simulink model "MINI_upgrade"  (R2021a)
settings: Solver=FixedStepAuto  StartTime=0.0  StopTime=10.0  FixedStep=0.001  RelTol=1e-3
InitFcn:
  | parameters;
model workspace: external: MATLAB File .\MINI_upgrade_DataFile.m (data not in the file)
values from neighbouring files (symbols this model uses):
  th10_ofst = -pi    (= -3.14159265359)    [parameters.m]
  th11_ofst = 0    [parameters.m]
  th12_ofst = pi    (= 3.14159265359)    [parameters.m]
  th13_ofst = 0    [parameters.m]
  th14_ofst = 0    [parameters.m]
  th15_ofst = 0    [parameters.m]
  th16_ofst = 0    [parameters.m]
  th1_ofst = pi/2    (= 1.57079632679)    [parameters.m]
  th2_ofst = -pi/2    (= -1.57079632679)    [parameters.m]
  th3_ofst = pi/2    (= 1.57079632679)    [parameters.m]
  th4_ofst = pi/2    (= 1.57079632679)    [parameters.m]
  th5_ofst = 0    [parameters.m]
  th6_ofst = 0    [parameters.m]
  th7_ofst = pi/2    (= 1.57079632679)    [parameters.m]
  th8_ofst = pi/2    (= 1.57079632679)    [parameters.m]
  th9_ofst = 0    [parameters.m]
undefined symbols (not defined in the file or in its folder): smiData, X, Y, Z
libraries: sm_lib x484, nesl_utility x17
(part 9 of 9)

== system MINI_upgrade/Upgraded_Body_1_RIGID/Copy_of_Upgraded_BodyUpgraded_Body_1_RIGID/Rivet_2_RIGID/River_01_1_RIGID ==
  ReferenceFrame : sm_lib/Frames and Transforms/Reference Frame
  Solid : sm_lib/Body Elements/File Solid  ExtGeomFileName=River_01_Default_sldprt.STEP  UnitType=FromFile  ExtGeomFileUnits=m  StepReaderType=HEX  ExportConvexHullGeometry=off  InertiaType=Custom  Mass=smiData.Solid(11).mass  MassUnits=kg  CenterOfMass=smiData.Solid(11).CoM  CenterOfMassUnits=mm  MomentsOfInertia=smiData.Solid(11).MoI  MomentsOfInertiaUnits=kg*mm^2  ProductsOfInertia=smiData.Solid(11).PoI  ProductsOfInertiaUnits=kg*mm^2  BasedOnType=DensityFromFile  Density=1000  DensityUnits=kg/m^3  DoExposeReferenceFrame=on  SerializedFrames=<Frames/>  GraphicType=FromGeometry  MarkerShape=Sphere  MarkerSize=10  GraphicVisPropType=SimpleVisualProperties  GraphicDiffuseColor=smiData.Solid(11).color  GraphicSpecularColor=[0.5 0.5 0.5 1.0]  GraphicAmbientColor=[0.15 0.15 0.15 1.0]  GraphicEmissiveColor=[0.0 0.0 0.0 1.0]  GraphicShininess=75  GraphicOpacity=smiData.Solid(11).opacity
  F : PMIOPort  Side=Left
  connections:
  Solid/RConn1 -- ReferenceFrame/RConn1 -- F/RConn1

== system MINI_upgrade/Upgraded_Body_1_RIGID/Copy_of_Upgraded_BodyUpgraded_Body_1_RIGID/Rivet_2_RIGID/River_02_1_RIGID ==
  ReferenceFrame : sm_lib/Frames and Transforms/Reference Frame
  Solid : sm_lib/Body Elements/File Solid  ExtGeomFileName=River_02_Default_sldprt.STEP  UnitType=FromFile  ExtGeomFileUnits=m  StepReaderType=HEX  ExportConvexHullGeometry=off  InertiaType=Custom  Mass=smiData.Solid(12).mass  MassUnits=kg  CenterOfMass=smiData.Solid(12).CoM  CenterOfMassUnits=mm  MomentsOfInertia=smiData.Solid(12).MoI  MomentsOfInertiaUnits=kg*mm^2  ProductsOfInertia=smiData.Solid(12).PoI  ProductsOfInertiaUnits=kg*mm^2  BasedOnType=DensityFromFile  Density=1000  DensityUnits=kg/m^3  DoExposeReferenceFrame=on  SerializedFrames=<Frames/>  GraphicType=FromGeometry  MarkerShape=Sphere  MarkerSize=10  GraphicVisPropType=SimpleVisualProperties  GraphicDiffuseColor=smiData.Solid(12).color  GraphicSpecularColor=[0.5 0.5 0.5 1.0]  GraphicAmbientColor=[0.15 0.15 0.15 1.0]  GraphicEmissiveColor=[0.0 0.0 0.0 1.0]  GraphicShininess=75  GraphicOpacity=smiData.Solid(12).opacity
  F : PMIOPort  Side=Left
  connections:
  Solid/RConn1 -- ReferenceFrame/RConn1 -- F/RConn1

== system MINI_upgrade/Upgraded_Body_1_RIGID/Copy_of_Upgraded_BodyUpgraded_Body_1_RIGID/Rivet_3_RIGID/River_01_1_RIGID ==
  ReferenceFrame : sm_lib/Frames and Transforms/Reference Frame
  Solid : sm_lib/Body Elements/File Solid  ExtGeomFileName=River_01_Default_sldprt.STEP  UnitType=FromFile  ExtGeomFileUnits=m  StepReaderType=HEX  ExportConvexHullGeometry=off  InertiaType=Custom  Mass=smiData.Solid(11).mass  MassUnits=kg  CenterOfMass=smiData.Solid(11).CoM  CenterOfMassUnits=mm  MomentsOfInertia=smiData.Solid(11).MoI  MomentsOfInertiaUnits=kg*mm^2  ProductsOfInertia=smiData.Solid(11).PoI  ProductsOfInertiaUnits=kg*mm^2  BasedOnType=DensityFromFile  Density=1000  DensityUnits=kg/m^3  DoExposeReferenceFrame=on  SerializedFrames=<Frames/>  GraphicType=FromGeometry  MarkerShape=Sphere  MarkerSize=10  GraphicVisPropType=SimpleVisualProperties  GraphicDiffuseColor=smiData.Solid(11).color  GraphicSpecularColor=[0.5 0.5 0.5 1.0]  GraphicAmbientColor=[0.15 0.15 0.15 1.0]  GraphicEmissiveColor=[0.0 0.0 0.0 1.0]  GraphicShininess=75  GraphicOpacity=smiData.Solid(11).opacity
  F : PMIOPort  Side=Left
  connections:
  Solid/RConn1 -- ReferenceFrame/RConn1 -- F/RConn1

== system MINI_upgrade/Upgraded_Body_1_RIGID/Copy_of_Upgraded_BodyUpgraded_Body_1_RIGID/Rivet_3_RIGID/River_02_1_RIGID ==
  ReferenceFrame : sm_lib/Frames and Transforms/Reference Frame
  Solid : sm_lib/Body Elements/File Solid  ExtGeomFileName=River_02_Default_sldprt.STEP  UnitType=FromFile  ExtGeomFileUnits=m  StepReaderType=HEX  ExportConvexHullGeometry=off  InertiaType=Custom  Mass=smiData.Solid(12).mass  MassUnits=kg  CenterOfMass=smiData.Solid(12).CoM  CenterOfMassUnits=mm  MomentsOfInertia=smiData.Solid(12).MoI  MomentsOfInertiaUnits=kg*mm^2  ProductsOfInertia=smiData.Solid(12).PoI  ProductsOfInertiaUnits=kg*mm^2  BasedOnType=DensityFromFile  Density=1000  DensityUnits=kg/m^3  DoExposeReferenceFrame=on  SerializedFrames=<Frames/>  GraphicType=FromGeometry  MarkerShape=Sphere  MarkerSize=10  GraphicVisPropType=SimpleVisualProperties  GraphicDiffuseColor=smiData.Solid(12).color  GraphicSpecularColor=[0.5 0.5 0.5 1.0]  GraphicAmbientColor=[0.15 0.15 0.15 1.0]  GraphicEmissiveColor=[0.0 0.0 0.0 1.0]  GraphicShininess=75  GraphicOpacity=smiData.Solid(12).opacity
  F : PMIOPort  Side=Left
  connections:
  Solid/RConn1 -- ReferenceFrame/RConn1 -- F/RConn1

== system MINI_upgrade/Upgraded_Body_1_RIGID/Copy_of_Upgraded_BodyUpgraded_Body_1_RIGID/Rivet_4_RIGID/River_01_1_RIGID ==
  ReferenceFrame : sm_lib/Frames and Transforms/Reference Frame
  Solid : sm_lib/Body Elements/File Solid  ExtGeomFileName=River_01_Default_sldprt.STEP  UnitType=FromFile  ExtGeomFileUnits=m  StepReaderType=HEX  ExportConvexHullGeometry=off  InertiaType=Custom  Mass=smiData.Solid(11).mass  MassUnits=kg  CenterOfMass=smiData.Solid(11).CoM  CenterOfMassUnits=mm  MomentsOfInertia=smiData.Solid(11).MoI  MomentsOfInertiaUnits=kg*mm^2  ProductsOfInertia=smiData.Solid(11).PoI  ProductsOfInertiaUnits=kg*mm^2  BasedOnType=DensityFromFile  Density=1000  DensityUnits=kg/m^3  DoExposeReferenceFrame=on  SerializedFrames=<Frames/>  GraphicType=FromGeometry  MarkerShape=Sphere  MarkerSize=10  GraphicVisPropType=SimpleVisualProperties  GraphicDiffuseColor=smiData.Solid(11).color  GraphicSpecularColor=[0.5 0.5 0.5 1.0]  GraphicAmbientColor=[0.15 0.15 0.15 1.0]  GraphicEmissiveColor=[0.0 0.0 0.0 1.0]  GraphicShininess=75  GraphicOpacity=smiData.Solid(11).opacity
  F : PMIOPort  Side=Left
  connections:
  Solid/RConn1 -- ReferenceFrame/RConn1 -- F/RConn1

== system MINI_upgrade/Upgraded_Body_1_RIGID/Copy_of_Upgraded_BodyUpgraded_Body_1_RIGID/Rivet_4_RIGID/River_02_1_RIGID ==
  ReferenceFrame : sm_lib/Frames and Transforms/Reference Frame
  Solid : sm_lib/Body Elements/File Solid  ExtGeomFileName=River_02_Default_sldprt.STEP  UnitType=FromFile  ExtGeomFileUnits=m  StepReaderType=HEX  ExportConvexHullGeometry=off  InertiaType=Custom  Mass=smiData.Solid(12).mass  MassUnits=kg  CenterOfMass=smiData.Solid(12).CoM  CenterOfMassUnits=mm  MomentsOfInertia=smiData.Solid(12).MoI  MomentsOfInertiaUnits=kg*mm^2  ProductsOfInertia=smiData.Solid(12).PoI  ProductsOfInertiaUnits=kg*mm^2  BasedOnType=DensityFromFile  Density=1000  DensityUnits=kg/m^3  DoExposeReferenceFrame=on  SerializedFrames=<Frames/>  GraphicType=FromGeometry  MarkerShape=Sphere  MarkerSize=10  GraphicVisPropType=SimpleVisualProperties  GraphicDiffuseColor=smiData.Solid(12).color  GraphicSpecularColor=[0.5 0.5 0.5 1.0]  GraphicAmbientColor=[0.15 0.15 0.15 1.0]  GraphicEmissiveColor=[0.0 0.0 0.0 1.0]  GraphicShininess=75  GraphicOpacity=smiData.Solid(12).opacity
  F : PMIOPort  Side=Left
  connections:
  Solid/RConn1 -- ReferenceFrame/RConn1 -- F/RConn1

== system MINI_upgrade/Upgraded_Body_1_RIGID/Body_v2_1_RIGID/Darwin_mini_bat_box_v2_1_RIGID/Darwin_mini_bat_box_stp_1_RIGID/DARWIN_MINI_LBB_040_stp_1_RIGID ==
  ReferenceFrame : sm_lib/Frames and Transforms/Reference Frame
  Solid : sm_lib/Body Elements/File Solid  ExtGeomFileName=DARWIN-MINI_LBB-040.stp_Default_sldprt.STEP  UnitType=FromFile  ExtGeomFileUnits=m  StepReaderType=HEX  ExportConvexHullGeometry=off  InertiaType=Custom  Mass=smiData.Solid(21).mass  MassUnits=kg  CenterOfMass=smiData.Solid(21).CoM  CenterOfMassUnits=mm  MomentsOfInertia=smiData.Solid(21).MoI  MomentsOfInertiaUnits=kg*mm^2  ProductsOfInertia=smiData.Solid(21).PoI  ProductsOfInertiaUnits=kg*mm^2  BasedOnType=DensityFromFile  Density=1000  DensityUnits=kg/m^3  DoExposeReferenceFrame=on  SerializedFrames=<Frames/>  GraphicType=FromGeometry  MarkerShape=Sphere  MarkerSize=10  GraphicVisPropType=SimpleVisualProperties  GraphicDiffuseColor=smiData.Solid(21).color  GraphicSpecularColor=[0.5 0.5 0.5 1.0]  GraphicAmbientColor=[0.15 0.15 0.15 1.0]  GraphicEmissiveColor=[0.0 0.0 0.0 1.0]  GraphicShininess=75  GraphicOpacity=smiData.Solid(21).opacity
  F : PMIOPort  Side=Left
  connections:
  Solid/RConn1 -- ReferenceFrame/RConn1 -- F/RConn1

== system MINI_upgrade/Upgraded_Body_1_RIGID/Body_v2_1_RIGID/Darwin_mini_bat_box_v2_1_RIGID/Darwin_mini_bat_box_stp_1_RIGID/DARWIN_MINI_LB_040_stp_1_RIGID ==
  ReferenceFrame : sm_lib/Frames and Transforms/Reference Frame
  Solid : sm_lib/Body Elements/File Solid  ExtGeomFileName=DARWIN-MINI_LB-040.stp_Default_sldprt.STEP  UnitType=FromFile  ExtGeomFileUnits=m  StepReaderType=HEX  ExportConvexHullGeometry=off  InertiaType=Custom  Mass=smiData.Solid(20).mass  MassUnits=kg  CenterOfMass=smiData.Solid(20).CoM  CenterOfMassUnits=mm  MomentsOfInertia=smiData.Solid(20).MoI  MomentsOfInertiaUnits=kg*mm^2  ProductsOfInertia=smiData.Solid(20).PoI  ProductsOfInertiaUnits=kg*mm^2  BasedOnType=DensityFromFile  Density=1000  DensityUnits=kg/m^3  DoExposeReferenceFrame=on  SerializedFrames=<Frames/>  GraphicType=FromGeometry  MarkerShape=Sphere  MarkerSize=10  GraphicVisPropType=SimpleVisualProperties  GraphicDiffuseColor=smiData.Solid(20).color  GraphicSpecularColor=[0.5 0.5 0.5 1.0]  GraphicAmbientColor=[0.15 0.15 0.15 1.0]  GraphicEmissiveColor=[0.0 0.0 0.0 1.0]  GraphicShininess=75  GraphicOpacity=smiData.Solid(20).opacity
  F : PMIOPort  Side=Left
  connections:
  Solid/RConn1 -- ReferenceFrame/RConn1 -- F/RConn1

== system MINI_upgrade/Upgraded_Body_1_RIGID/Body_v2_1_RIGID/Darwin_mini_bat_box_v2_2_RIGID/Darwin_mini_bat_box_stp_1_RIGID/DARWIN_MINI_LBB_040_stp_1_RIGID ==
  ReferenceFrame : sm_lib/Frames and Transforms/Reference Frame
  Solid : sm_lib/Body Elements/File Solid  ExtGeomFileName=DARWIN-MINI_LBB-040.stp_Default_sldprt.STEP  UnitType=FromFile  ExtGeomFileUnits=m  StepReaderType=HEX  ExportConvexHullGeometry=off  InertiaType=Custom  Mass=smiData.Solid(21).mass  MassUnits=kg  CenterOfMass=smiData.Solid(21).CoM  CenterOfMassUnits=mm  MomentsOfInertia=smiData.Solid(21).MoI  MomentsOfInertiaUnits=kg*mm^2  ProductsOfInertia=smiData.Solid(21).PoI  ProductsOfInertiaUnits=kg*mm^2  BasedOnType=DensityFromFile  Density=1000  DensityUnits=kg/m^3  DoExposeReferenceFrame=on  SerializedFrames=<Frames/>  GraphicType=FromGeometry  MarkerShape=Sphere  MarkerSize=10  GraphicVisPropType=SimpleVisualProperties  GraphicDiffuseColor=smiData.Solid(21).color  GraphicSpecularColor=[0.5 0.5 0.5 1.0]  GraphicAmbientColor=[0.15 0.15 0.15 1.0]  GraphicEmissiveColor=[0.0 0.0 0.0 1.0]  GraphicShininess=75  GraphicOpacity=smiData.Solid(21).opacity
  F : PMIOPort  Side=Left
  connections:
  Solid/RConn1 -- ReferenceFrame/RConn1 -- F/RConn1

== system MINI_upgrade/Upgraded_Body_1_RIGID/Body_v2_1_RIGID/Darwin_mini_bat_box_v2_2_RIGID/Darwin_mini_bat_box_stp_1_RIGID/DARWIN_MINI_LB_040_stp_1_RIGID ==
  ReferenceFrame : sm_lib/Frames and Transforms/Reference Frame
  Solid : sm_lib/Body Elements/File Solid  ExtGeomFileName=DARWIN-MINI_LB-040.stp_Default_sldprt.STEP  UnitType=FromFile  ExtGeomFileUnits=m  StepReaderType=HEX  ExportConvexHullGeometry=off  InertiaType=Custom  Mass=smiData.Solid(20).mass  MassUnits=kg  CenterOfMass=smiData.Solid(20).CoM  CenterOfMassUnits=mm  MomentsOfInertia=smiData.Solid(20).MoI  MomentsOfInertiaUnits=kg*mm^2  ProductsOfInertia=smiData.Solid(20).PoI  ProductsOfInertiaUnits=kg*mm^2  BasedOnType=DensityFromFile  Density=1000  DensityUnits=kg/m^3  DoExposeReferenceFrame=on  SerializedFrames=<Frames/>  GraphicType=FromGeometry  MarkerShape=Sphere  MarkerSize=10  GraphicVisPropType=SimpleVisualProperties  GraphicDiffuseColor=smiData.Solid(20).color  GraphicSpecularColor=[0.5 0.5 0.5 1.0]  GraphicAmbientColor=[0.15 0.15 0.15 1.0]  GraphicEmissiveColor=[0.0 0.0 0.0 1.0]  GraphicShininess=75  GraphicOpacity=smiData.Solid(20).opacity
  F : PMIOPort  Side=Left
  connections:
  Solid/RConn1 -- ReferenceFrame/RConn1 -- F/RConn1

== matlab function MINI_upgrade/MATLAB Function1 ==
  data: x_RH_in input; th1 output; y_RH_in input; z_RH_in input; th3 output; th5 output
% ECE 598 JK Fall 2020 University of Illinois at Urbana-Champaign
% ROBOTIS MINI Right Hand Inverse Kinematics
% 09/07/2020 by Kevin Gim (kggim2@illinois.edu)

function [th1,th3,th5] = IK_RH(x_RH_in, y_RH_in, z_RH_in)

L_sh = 39; % Origin to arm roll joint
L_a1 = 18; % Shoulder bracket horizontal distance
L_a2 = 12; % Shoulder bracket vertical distance
L_a3 = 45; % Upper arm length
L_a4 = 72; % Lower arm length

% Position of Right hand in Initial Pose (all the right arm motor angle == 0)

th1 = 0;
th3 = 0;
th5 = 0;


% Right Arm
x_RH = x_RH_in;
y_RH = y_RH_in;
z_RH = z_RH_in;
x_RH0 = x_RH;
y_RH0 = y_RH + (L_sh + L_a1);
z_RH0 = z_RH;

th1 = -atan(x_RH0/(z_RH0+0.00001));

% Range of XL320 motor -150 to 150 deg
if (th1 > 2.618)
    th1 = 2.618;
elseif (th1 < -2.618)
    th1 = -2.618;
else
    th1 = th1;
end

R1_RH = sqrt((x_RH0 - L_a2*sin(th1))^2 + y_RH0^2 + (z_RH0 + L_a2*cos(th1))^2);

if (R1_RH > 117)
    R1_RH = 117
else
    R1_RH = R1_RH;
end

alpha_RH = acos((L_a3^2 + L_a4^2 -R1_RH^2)/(2*L_a3*L_a4));

% Elbow Joint angle
th5 = -pi + alpha_RH;
R2_RH = sqrt((x_RH0 - L_a2*sin(th1))^2 + (z_RH0 + L_a2*cos(th1))^2);

% Shoulder Joint angle
if (z_RH > 0)
th3 = pi/2 + (atan(y_RH0/R2_RH) + acos((L_a3^2 + R1_RH^2 - L_a4^2)/(2*L_a3*R1_RH)));
else
th3 = -pi/2 + (-atan(y_RH0/R2_RH) + acos((L_a3^2 + R1_RH^2 - L_a4^2)/(2*L_a3*R1_RH)));
end

== matlab function MINI_upgrade/MATLAB Function2 ==
  data: x_LH_in input; th2 output; th4 output; th6 output; y_LH_in input; z_LH_in input
% ECE 598 JK Fall 2020 University of Illinois at Urbana-Champaign
% ROBOTIS MINI Left Hand Inverse Kinematics
% 09/07/2020 by Kevin Gim (kggim2@illinois.edu)


function [th2,th4,th6] = IK_LH(x_LH_in, y_LH_in, z_LH_in)

L_sh = 39; % Origin to arm roll joint
L_a1 = 18; % Shoulder bracket horizontal distance
L_a2 = 12; % Shoulder bracket vertical distance
L_a3 = 45; % Upper arm length
L_a4 = 72; % Lower arm length


th2 = 0;
th4 = 0;
th6 = 0;

% Left Arm
x_LH = x_LH_in;
y_LH = y_LH_in;
z_LH = z_LH_in;

x_LH0 = x_LH;
y_LH0 = y_LH - (L_sh + L_a1);
z_LH0 = z_LH;

th2 = atan(x_LH0/(z_LH0+0.00001));

% Range of XL320 motor -150 to 150 deg
if (th2 > 2.618)
    th2 = 2.618;
elseif (th2 < -2.618)
    th2 = -2.618;
else
    th2 = th2;
end

R1_LH = sqrt((x_LH0 - L_a2*sin(th2))^2 + y_LH0^2 + (z_LH0+L_a2*cos(th2))^2);

if (R1_LH > 117)
    R1_LH = 117;
else
    R1_LH = R1_LH;
end

alpha_LH = acos((L_a3^2 + L_a4^2 -R1_LH^2)/(2*L_a3*L_a4));

% Elbow Joint angle 
th6 = pi - alpha_LH;

R2_LH = sqrt((x_LH0 - L_a2*sin(th2))^2 + (z_LH0 + L_a2*cos(th2))^2);

% Shoulder Joint angle
if (z_LH0 > 0)
    th4 = -((atan(R2_LH/y_LH0) + acos((L_a3^2 + R1_LH^2 - L_a4^2)/(2*L_a3*R1_LH))));
else
    th4 = -(-pi/2 + (atan(y_LH0/R2_LH) + acos((L_a3^2 + R1_LH^2 - L_a4^2)/(2*L_a3*R1_LH))));
end

== matlab function MINI_upgrade/MATLAB Function ==
  data: x_LF_in input; th8 output; y_LF_in input; z_LF_in input; roll_LF input; pitch_LF input; th10 output; th12 output; th14 output; th16 output
% ECE 598 JK Fall 2020 University of Illinois at Urbana-Champaign
% ROBOTIS MINI Left Foot Inverse Kinematics
% 09/07/2020 by Kevin Gim (kggim2@illinois.edu)

function [th8, th10, th12, th14, th16] = IK_LF(x_LF_in, y_LF_in, z_LF_in, roll_LF, pitch_LF)

%Left foot
% Controllable position x, y, z, roll, pitch

L_by = 24; % Origin to pelvis vertical length
L_bz = 72; % Pelvis horizontal length
L_bx = 15; % Shoulder joint axis to Leg center (On Sagittal Plane)
L_l1 = 6;  % Pelvis Roll axis to pitch axis
L_l2 = 45; % Thigh Length
L_l3 = 42; % Shank Length
L_l4 = 31;  % Ankle Length
L_f = 9; % Foot horizontal length

x_LF = x_LF_in;
y_LF = y_LF_in;
z_LF = z_LF_in;


R0LF = RX(roll_LF) * RY(pitch_LF);
T0LF = R0LF + TXYZ(x_LF, y_LF, z_LF) - eye(4);
T016 = T0LF * RY(-(pi)/2) *RZ((pi)) * TXYZ(-L_l4,L_f,0);
TLF0_16 = (TXYZ(L_bx,L_by,-L_bz)*RY((pi)/2))\T016;
pos_LF = TLF0_16(1:3,4);

th8 = atan(pos_LF(2)/pos_LF(1));
R1_LF = sqrt((pos_LF(1)-L_l1*cos(th8))^2 + (pos_LF(2)-L_l1*sin(th8))^2 + pos_LF(3)^2);
alpha_LF = acos((L_l2^2 + L_l3^2 -R1_LF^2)/(2*L_l2*L_l3));

th12 = -pi+alpha_LF;
R2_LF = sqrt((pos_LF(1)-L_l1*cos(th8))^2 + (pos_LF(2)-L_l1*sin(th8))^2);

th10 = (atan(pos_LF(3)/R2_LF) + acos((L_l2^2 + R1_LF^2 - L_l3^2)/(2*L_l2*R1_LF)));


T_LF0_12 = [ cos(th10 + th12)*cos(th8), -sin(th10 + th12)*cos(th8),  sin(th8), cos(th8)*(L_l1 + L_l2*cos(th10));
    cos(th10 + th12)*sin(th8), -sin(th10 + th12)*sin(th8), -cos(th8), sin(th8)*(L_l1 + L_l2*cos(th10));
    sin(th10 + th12),           cos(th10 + th12),         0,                   L_l2*sin(th10);
    0,                          0,         0,                                1];

T_12_16 = (T_LF0_12)\TLF0_16;
th14 = -asin(T_12_16(1,3));
th16 = -asin(-T_12_16(3,1));

== matlab function MINI_upgrade/MATLAB Function3 ==
  data: x_RF_in input; th7 output; y_RF_in input; z_RF_in input; roll_RF input; pitch_RF input; th9 output; th11 output; th13 output; th15 output
% ECE 598 JK Fall 2020 University of Illinois at Urbana-Champaign
% ROBOTIS MINI Right Foot Inverse Kinematics
% 09/07/2020 by Kevin Gim (kggim2@illinois.edu)

function [th7,th9, th11, th13, th15] = IK_RF(x_RF_in, y_RF_in, z_RF_in, roll_RF, pitch_RF)

% Right foot
% Controllable position x, y, z, roll, pitch

L_by = 24; % Origin to pelvis vertical length
L_bz = 72; % Pelvis horizontal length
L_bx = 15; % Shoulder joint axis to Leg center (On Sagittal Plane)
L_l1 = 6;  % Pelvis Roll axis to pitch axis
L_l2 = 45; % Thigh Length
L_l3 = 42; % Shank Length
L_l4 = 31;  % Ankle Length
L_f = 9; % Foot horizontal length

x_RF = x_RF_in;
y_RF = y_RF_in;
z_RF = z_RF_in;



R0RF = RX(roll_RF) * RY(pitch_RF);
T0RF = R0RF + TXYZ(x_RF, y_RF, z_RF) - eye(4);
T015 = T0RF * RY(-(pi)/2) * RZ((pi)) * TXYZ(-L_l4,-L_f,0);
TRF0_15 = (TXYZ(L_bx,-L_by,-L_bz)*RY((pi)/2))\T015;

pos_RF = TRF0_15(1:3,4);
th7 = atan(pos_RF(2)/pos_RF(1));
R1_RF = sqrt((pos_RF(1)-L_l1*cos(th7))^2 + (pos_RF(2)-L_l1*sin(th7))^2 + pos_RF(3)^2);
alpha_RF = acos((L_l2^2 + L_l3^2 -R1_RF^2)/(2*L_l2*L_l3));
th11 = pi-alpha_RF;
R2_RF = sqrt((pos_RF(1)-L_l1*cos(th7))^2 + (pos_RF(2)-L_l1*sin(th7))^2);

th9 = -((atan(pos_RF(3)/R2_RF) + acos((L_l2^2 + R1_RF^2 - L_l3^2)/(2*L_l2*R1_RF))));

T_RF0_11 = [ cos(th9 + th11)*cos(th7), -sin(th9 + th11)*cos(th7), -sin(th7), cos(th7)*(L_l1 + L_l2*cos(th9));
    cos(th9 + th11)*sin(th7), -sin(th9 + th11)*sin(th7),  cos(th7), sin(th7)*(L_l1 + L_l2*cos(th9));
    -sin(th9 + th11),          -cos(th9 + th11),         0,                  -L_l2*sin(th9);
    0,                         0,         0,                               1];

T_11_15 = (T_RF0_11)\TRF0_15;
th13 = asin(T_11_15(1,3));
th15 = asin(-T_11_15(3,1));
